simulink model "transPriority"  (R2012b)
settings: Solver=ode45  StartTime=0.0  StopTime=inf  RelTol=1e-3
settings Model: Creator=jrivitus  LastModifiedBy=jrivitus
settings DebuggingCC: ParameterPrecisionLossMsg=none  FcnCallInpInsideContextMsg=UseLocalSettings  StrictBusMsg=Warning
settings SFSimCC: SimParseCustomCode=off
settings GRTTargetCC: CombineOutputUpdateFcns=off  GRTInterface=on

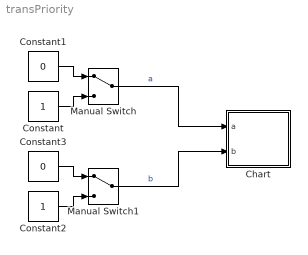
== system transPriority ==
  Chart : Stateflow chart  TreatAsAtomicUnit=on
  Constant : Constant
  Constant1 : Constant  Value=0
  Constant2 : Constant
  Constant3 : Constant  Value=0
  Manual Switch : ManualSwitch
  Manual Switch1 : ManualSwitch
  wires:
  Constant1/1 -> Manual Switch/1
  Constant/1 -> Manual Switch/2
  Manual Switch/1 -> Chart/1(a)  "a"
  Constant3/1 -> Manual Switch1/1
  Constant2/1 -> Manual Switch1/2
  Manual Switch1/1 -> Chart/2(b)  "b"

== stateflow chart transPriority/Chart ==
  (default) -> (junction 2)
  (junction 2) -> (junction 3) [order 1] : [b>0]
  (junction 2) -> (junction 4) [order 2] : [a>0]
  (junction 3) -> (junction 5)
  (junction 4) -> (junction 5)
  (junction 2) -> (junction 5) [order 3]
  data: a input; b input
